simulink model "lab4"  (R2024a)
settings: Solver=VariableStepAuto  StartTime=0.0  StopTime=1  RelTol=1e-3
model workspace (MAT data in the model file):
  ampl = 1
  delta_f = 100
  delta_fc = 4000
  fd = 1024000
undefined symbols (not defined in the file): fdesignblkfcn, gcbh
libraries: dsparch4 x13, commanapbnd3 x13, dspsrcs4 x12, dspfdesign x1
settings Model: Creator=Egor Masterskikh  LastModifiedBy=Egor Masterskikh

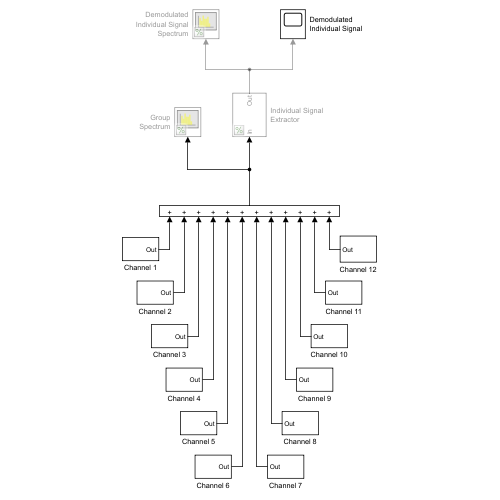
[thumbnail: Simulink's stored preview of the top-level diagram]
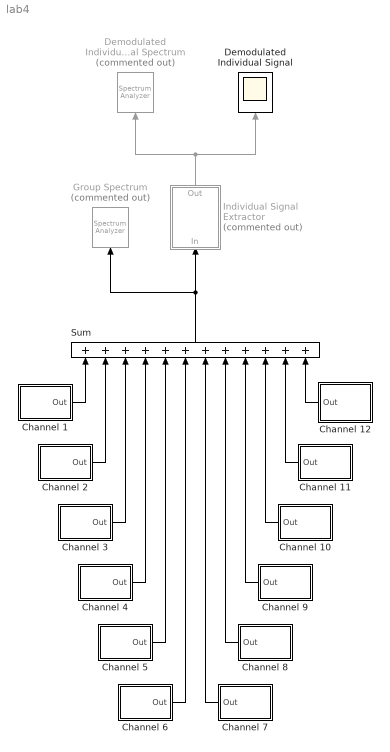
== system lab4 ==
  Channel 1 : Subsystem  mask{f=900, fc=64000}
      mask prompts: f "Frequency (Hz)"; fc "Carrier frequency (Hz)"
  Channel 10 : Subsystem  mask{f=1800, fc=100000}
      mask prompts: f "Frequency (Hz)"; fc "Carrier frequency (Hz)"
  Channel 11 : Subsystem  mask{f=1900, fc=104000}
      mask prompts: f "Frequency (Hz)"; fc "Carrier frequency (Hz)"
  Channel 12 : Subsystem  mask{f=2000, fc=108000}
      mask prompts: f "Frequency (Hz)"; fc "Carrier frequency (Hz)"
  Channel 2 : Subsystem  mask{f=1000, fc=68000}
      mask prompts: f "Frequency (Hz)"; fc "Carrier frequency (Hz)"
  Channel 3 : Subsystem  mask{f=1100, fc=72000}
      mask prompts: f "Frequency (Hz)"; fc "Carrier frequency (Hz)"
  Channel 4 : Subsystem  mask{f=1200, fc=76000}
      mask prompts: f "Frequency (Hz)"; fc "Carrier frequency (Hz)"
  Channel 5 : Subsystem  mask{f=1300, fc=80000}
      mask prompts: f "Frequency (Hz)"; fc "Carrier frequency (Hz)"
  Channel 6 : Subsystem  mask{f=1400, fc=84000}
      mask prompts: f "Frequency (Hz)"; fc "Carrier frequency (Hz)"
  Channel 7 : Subsystem  mask{f=1500, fc=88000}
      mask prompts: f "Frequency (Hz)"; fc "Carrier frequency (Hz)"
  Channel 8 : Subsystem  mask{f=1600, fc=92000}
      mask prompts: f "Frequency (Hz)"; fc "Carrier frequency (Hz)"
  Channel 9 : Subsystem  mask{f=1700, fc=96000}
      mask prompts: f "Frequency (Hz)"; fc "Carrier frequency (Hz)"
  Demodulated Individual Signal : Scope
  Demodulated Individual Signal Spectrum : SpectrumAnalyzer  Commented=on  WindowPosition=[154.000000,73.000000,765.000000,744.000000,]  ScopeFrameLocation=window  SampleRate=44.1e3  PlotAsTwoSidedSpectrum=off  FrequencySpan=Start and stop frequencies  StartFrequency=50  YLimits=[-52.2671399,38.98350768]  SelectedToolstripTab=spectrumAnalyzerToolstrip.estimationTab
  Group Spectrum : SpectrumAnalyzer  Commented=on  WindowPosition=[318.000000,220.000000,765.000000,500.000000,]  ScopeFrameLocation=window  SampleRate=44.1e3  PlotAsTwoSidedSpectrum=off  StartFrequency=20  StopFrequency=20e3  YLimits=[-282.95043207,54.73793571]
  Individual Signal Extractor : Subsystem  Commented=on  mask{ch_num=1, fc=64000, f_cutoff=64100}
      mask prompts: ch_num "Extracted channel number"; fc "Carrier frequency (Hz)"; f_cutoff "Cutoff frequency (Hz)"
  Sum : Sum  Inputs=++++++++++++
  wires:
  Sum/1 -> Group Spectrum/1, Individual Signal Extractor/1(In)
  Channel 1/1(Out) -> Sum/1
  Individual Signal Extractor/1(Out) -> Demodulated Individual Signal/1, Demodulated Individual Signal Spectrum/1
  Channel 12/1(Out) -> Sum/12
  Channel 2/1(Out) -> Sum/2
  Channel 3/1(Out) -> Sum/3
  Channel 4/1(Out) -> Sum/4
  Channel 11/1(Out) -> Sum/11
  Channel 10/1(Out) -> Sum/10
  Channel 9/1(Out) -> Sum/9
  Channel 5/1(Out) -> Sum/5
  Channel 8/1(Out) -> Sum/8
  Channel 6/1(Out) -> Sum/6
  Channel 7/1(Out) -> Sum/7

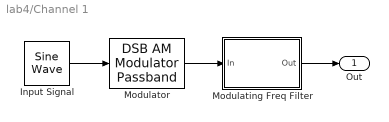
== system lab4/Channel 1 ==
  Input Signal : dspsrcs4/Sine Wave  Amplitude=ampl  Frequency=f  Phase=0  SampleMode=Discrete  OutComplex=Real  CompMethod=Trigonometric fcn  TableSize=Speed  SampleTime=1 / fd  SamplesPerFrame=1  ResetState=Restart at time zero  OutputFrames=off  dataType=double  wordLen=16  udDataType=sfix(16)  fracBitsMode=Best precision  numFracBits=15  OutDataTypeStr=double  LastOutDataTypeStr=double
  Modulating Freq Filter : Subsystem  DialogController=fdesignblkfcn  InitFcn=fdesignblkfcn(gcbh, {'InitFcn'});  mask(Bandpass Filter){}
      mask help: dsp:DSPFilterDesignBlockDialog:BandpassFdesign_MaskDesc
      settings: CopyFcn=fdesignblkfcn(gcbh, {'CopyFcn'});
      mask Help: helpview(mapfilelocation('dsp'), 'dspbandpassfilter');
      mask Display: disp('Bandpass');
  Modulator : commanapbnd3/DSB AM Modulator Passband  Fc=fc  Ph=0  Offset=ampl
  Out : Outport
  wires:
  Modulator/1 -> Modulating Freq Filter/1(In)
  Input Signal/1 -> Modulator/1
  Modulating Freq Filter/1(Out) -> Out/1

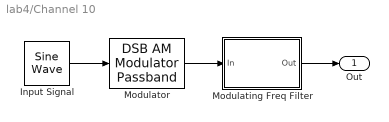
== system lab4/Channel 10 ==
  Input Signal : dspsrcs4/Sine Wave  Amplitude=ampl  Frequency=f  Phase=0  SampleMode=Discrete  OutComplex=Real  CompMethod=Trigonometric fcn  TableSize=Speed  SampleTime=1 / fd  SamplesPerFrame=1  ResetState=Restart at time zero  OutputFrames=off  dataType=double  wordLen=16  udDataType=sfix(16)  fracBitsMode=Best precision  numFracBits=15  OutDataTypeStr=double  LastOutDataTypeStr=double
  Modulating Freq Filter : Subsystem  DialogController=fdesignblkfcn  InitFcn=fdesignblkfcn(gcbh, {'InitFcn'});  mask(Bandpass Filter){}
      mask help: dsp:DSPFilterDesignBlockDialog:BandpassFdesign_MaskDesc
      settings: CopyFcn=fdesignblkfcn(gcbh, {'CopyFcn'});
      mask Help: helpview(mapfilelocation('dsp'), 'dspbandpassfilter');
      mask Display: disp('Bandpass');
  Modulator : commanapbnd3/DSB AM Modulator Passband  Fc=fc  Ph=0  Offset=ampl
  Out : Outport
  wires:
  Modulator/1 -> Modulating Freq Filter/1(In)
  Input Signal/1 -> Modulator/1
  Modulating Freq Filter/1(Out) -> Out/1

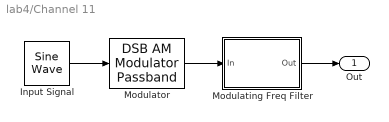
== system lab4/Channel 11 ==
  Input Signal : dspsrcs4/Sine Wave  Amplitude=ampl  Frequency=f  Phase=0  SampleMode=Discrete  OutComplex=Real  CompMethod=Trigonometric fcn  TableSize=Speed  SampleTime=1 / fd  SamplesPerFrame=1  ResetState=Restart at time zero  OutputFrames=off  dataType=double  wordLen=16  udDataType=sfix(16)  fracBitsMode=Best precision  numFracBits=15  OutDataTypeStr=double  LastOutDataTypeStr=double
  Modulating Freq Filter : Subsystem  DialogController=fdesignblkfcn  InitFcn=fdesignblkfcn(gcbh, {'InitFcn'});  mask(Bandpass Filter){}
      mask help: dsp:DSPFilterDesignBlockDialog:BandpassFdesign_MaskDesc
      settings: CopyFcn=fdesignblkfcn(gcbh, {'CopyFcn'});
      mask Help: helpview(mapfilelocation('dsp'), 'dspbandpassfilter');
      mask Display: disp('Bandpass');
  Modulator : commanapbnd3/DSB AM Modulator Passband  Fc=fc  Ph=0  Offset=ampl
  Out : Outport
  wires:
  Modulator/1 -> Modulating Freq Filter/1(In)
  Input Signal/1 -> Modulator/1
  Modulating Freq Filter/1(Out) -> Out/1

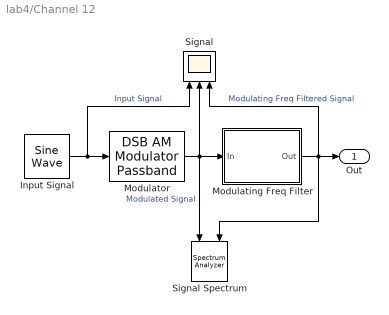
== system lab4/Channel 12 ==
  Input Signal : dspsrcs4/Sine Wave  Amplitude=ampl  Frequency=f  Phase=0  SampleMode=Discrete  OutComplex=Real  CompMethod=Trigonometric fcn  TableSize=Speed  SampleTime=1 / fd  SamplesPerFrame=1  ResetState=Restart at time zero  OutputFrames=off  dataType=double  wordLen=16  udDataType=sfix(16)  fracBitsMode=Best precision  numFracBits=15  OutDataTypeStr=double  LastOutDataTypeStr=double
  Modulating Freq Filter : Subsystem  DialogController=fdesignblkfcn  InitFcn=fdesignblkfcn(gcbh, {'InitFcn'});  mask(Bandpass Filter){}
      mask help: dsp:DSPFilterDesignBlockDialog:BandpassFdesign_MaskDesc
      settings: CopyFcn=fdesignblkfcn(gcbh, {'CopyFcn'});
      mask Help: helpview(mapfilelocation('dsp'), 'dspbandpassfilter');
      mask Display: disp('Bandpass');
  Modulator : commanapbnd3/DSB AM Modulator Passband  Fc=fc  Ph=0  Offset=ampl
  Signal : Scope  NumInputPorts=3
  Signal Spectrum : SpectrumAnalyzer  NumInputPorts=2  WindowPosition=[625.000000,219.000000,459.000000,419.000000,]  Visible=on  ScopeFrameLocation=window  SampleRate=1024000  PlotAsTwoSidedSpectrum=off  FrequencySpan=Start and stop frequencies  StartFrequency=102000  StopFrequency=116000  YLimits=[-95.72814975,34.95307911]  ShowLegend=on  SelectedToolstripTab=spectrumAnalyzerToolstrip.estimationTab
  Out : Outport
  wires:
  Modulator/1 -> Signal Spectrum/1, Signal/2, Modulating Freq Filter/1(In)  "Modulated Signal"
  Input Signal/1 -> Modulator/1, Signal/1  "Input Signal"
  Modulating Freq Filter/1(Out) -> Signal/3, Signal Spectrum/2, Out/1  "Modulating Freq Filtered Signal"

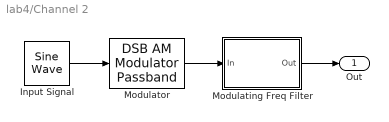
== system lab4/Channel 2 ==
  Input Signal : dspsrcs4/Sine Wave  Amplitude=ampl  Frequency=f  Phase=0  SampleMode=Discrete  OutComplex=Real  CompMethod=Trigonometric fcn  TableSize=Speed  SampleTime=1 / fd  SamplesPerFrame=1  ResetState=Restart at time zero  OutputFrames=off  dataType=double  wordLen=16  udDataType=sfix(16)  fracBitsMode=Best precision  numFracBits=15  OutDataTypeStr=double  LastOutDataTypeStr=double
  Modulating Freq Filter : Subsystem  DialogController=fdesignblkfcn  InitFcn=fdesignblkfcn(gcbh, {'InitFcn'});  mask(Bandpass Filter){}
      mask help: dsp:DSPFilterDesignBlockDialog:BandpassFdesign_MaskDesc
      settings: CopyFcn=fdesignblkfcn(gcbh, {'CopyFcn'});
      mask Help: helpview(mapfilelocation('dsp'), 'dspbandpassfilter');
      mask Display: disp('Bandpass');
  Modulator : commanapbnd3/DSB AM Modulator Passband  Fc=fc  Ph=0  Offset=ampl
  Out : Outport
  wires:
  Modulator/1 -> Modulating Freq Filter/1(In)
  Input Signal/1 -> Modulator/1
  Modulating Freq Filter/1(Out) -> Out/1

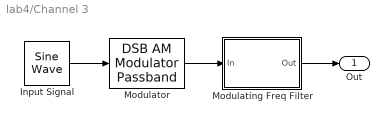
== system lab4/Channel 3 ==
  Input Signal : dspsrcs4/Sine Wave  Amplitude=ampl  Frequency=f  Phase=0  SampleMode=Discrete  OutComplex=Real  CompMethod=Trigonometric fcn  TableSize=Speed  SampleTime=1 / fd  SamplesPerFrame=1  ResetState=Restart at time zero  OutputFrames=off  dataType=double  wordLen=16  udDataType=sfix(16)  fracBitsMode=Best precision  numFracBits=15  OutDataTypeStr=double  LastOutDataTypeStr=double
  Modulating Freq Filter : Subsystem  DialogController=fdesignblkfcn  InitFcn=fdesignblkfcn(gcbh, {'InitFcn'});  mask(Bandpass Filter){}
      mask help: dsp:DSPFilterDesignBlockDialog:BandpassFdesign_MaskDesc
      settings: CopyFcn=fdesignblkfcn(gcbh, {'CopyFcn'});
      mask Help: helpview(mapfilelocation('dsp'), 'dspbandpassfilter');
      mask Display: disp('Bandpass');
  Modulator : commanapbnd3/DSB AM Modulator Passband  Fc=fc  Ph=0  Offset=ampl
  Out : Outport
  wires:
  Modulator/1 -> Modulating Freq Filter/1(In)
  Input Signal/1 -> Modulator/1
  Modulating Freq Filter/1(Out) -> Out/1

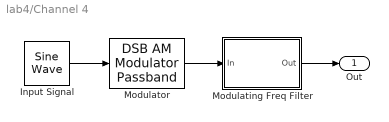
== system lab4/Channel 4 ==
  Input Signal : dspsrcs4/Sine Wave  Amplitude=ampl  Frequency=f  Phase=0  SampleMode=Discrete  OutComplex=Real  CompMethod=Trigonometric fcn  TableSize=Speed  SampleTime=1 / fd  SamplesPerFrame=1  ResetState=Restart at time zero  OutputFrames=off  dataType=double  wordLen=16  udDataType=sfix(16)  fracBitsMode=Best precision  numFracBits=15  OutDataTypeStr=double  LastOutDataTypeStr=double
  Modulating Freq Filter : Subsystem  DialogController=fdesignblkfcn  InitFcn=fdesignblkfcn(gcbh, {'InitFcn'});  mask(Bandpass Filter){}
      mask help: dsp:DSPFilterDesignBlockDialog:BandpassFdesign_MaskDesc
      settings: CopyFcn=fdesignblkfcn(gcbh, {'CopyFcn'});
      mask Help: helpview(mapfilelocation('dsp'), 'dspbandpassfilter');
      mask Display: disp('Bandpass');
  Modulator : commanapbnd3/DSB AM Modulator Passband  Fc=fc  Ph=0  Offset=ampl
  Out : Outport
  wires:
  Modulator/1 -> Modulating Freq Filter/1(In)
  Input Signal/1 -> Modulator/1
  Modulating Freq Filter/1(Out) -> Out/1

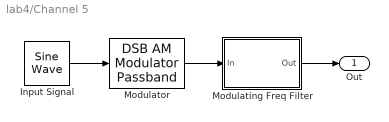
== system lab4/Channel 5 ==
  Input Signal : dspsrcs4/Sine Wave  Amplitude=ampl  Frequency=f  Phase=0  SampleMode=Discrete  OutComplex=Real  CompMethod=Trigonometric fcn  TableSize=Speed  SampleTime=1 / fd  SamplesPerFrame=1  ResetState=Restart at time zero  OutputFrames=off  dataType=double  wordLen=16  udDataType=sfix(16)  fracBitsMode=Best precision  numFracBits=15  OutDataTypeStr=double  LastOutDataTypeStr=double
  Modulating Freq Filter : Subsystem  DialogController=fdesignblkfcn  InitFcn=fdesignblkfcn(gcbh, {'InitFcn'});  mask(Bandpass Filter){}
      mask help: dsp:DSPFilterDesignBlockDialog:BandpassFdesign_MaskDesc
      settings: CopyFcn=fdesignblkfcn(gcbh, {'CopyFcn'});
      mask Help: helpview(mapfilelocation('dsp'), 'dspbandpassfilter');
      mask Display: disp('Bandpass');
  Modulator : commanapbnd3/DSB AM Modulator Passband  Fc=fc  Ph=0  Offset=ampl
  Out : Outport
  wires:
  Modulator/1 -> Modulating Freq Filter/1(In)
  Input Signal/1 -> Modulator/1
  Modulating Freq Filter/1(Out) -> Out/1

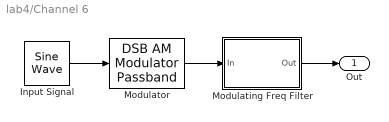
== system lab4/Channel 6 ==
  Input Signal : dspsrcs4/Sine Wave  Amplitude=ampl  Frequency=f  Phase=0  SampleMode=Discrete  OutComplex=Real  CompMethod=Trigonometric fcn  TableSize=Speed  SampleTime=1 / fd  SamplesPerFrame=1  ResetState=Restart at time zero  OutputFrames=off  dataType=double  wordLen=16  udDataType=sfix(16)  fracBitsMode=Best precision  numFracBits=15  OutDataTypeStr=double  LastOutDataTypeStr=double
  Modulating Freq Filter : Subsystem  DialogController=fdesignblkfcn  InitFcn=fdesignblkfcn(gcbh, {'InitFcn'});  mask(Bandpass Filter){}
      mask help: dsp:DSPFilterDesignBlockDialog:BandpassFdesign_MaskDesc
      settings: CopyFcn=fdesignblkfcn(gcbh, {'CopyFcn'});
      mask Help: helpview(mapfilelocation('dsp'), 'dspbandpassfilter');
      mask Display: disp('Bandpass');
  Modulator : commanapbnd3/DSB AM Modulator Passband  Fc=fc  Ph=0  Offset=ampl
  Out : Outport
  wires:
  Modulator/1 -> Modulating Freq Filter/1(In)
  Input Signal/1 -> Modulator/1
  Modulating Freq Filter/1(Out) -> Out/1

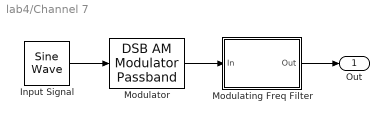
== system lab4/Channel 7 ==
  Input Signal : dspsrcs4/Sine Wave  Amplitude=ampl  Frequency=f  Phase=0  SampleMode=Discrete  OutComplex=Real  CompMethod=Trigonometric fcn  TableSize=Speed  SampleTime=1 / fd  SamplesPerFrame=1  ResetState=Restart at time zero  OutputFrames=off  dataType=double  wordLen=16  udDataType=sfix(16)  fracBitsMode=Best precision  numFracBits=15  OutDataTypeStr=double  LastOutDataTypeStr=double
  Modulating Freq Filter : Subsystem  DialogController=fdesignblkfcn  InitFcn=fdesignblkfcn(gcbh, {'InitFcn'});  mask(Bandpass Filter){}
      mask help: dsp:DSPFilterDesignBlockDialog:BandpassFdesign_MaskDesc
      settings: CopyFcn=fdesignblkfcn(gcbh, {'CopyFcn'});
      mask Help: helpview(mapfilelocation('dsp'), 'dspbandpassfilter');
      mask Display: disp('Bandpass');
  Modulator : commanapbnd3/DSB AM Modulator Passband  Fc=fc  Ph=0  Offset=ampl
  Out : Outport
  wires:
  Modulator/1 -> Modulating Freq Filter/1(In)
  Input Signal/1 -> Modulator/1
  Modulating Freq Filter/1(Out) -> Out/1

== system lab4/Channel 8 ==
  Input Signal : dspsrcs4/Sine Wave  Amplitude=ampl  Frequency=f  Phase=0  SampleMode=Discrete  OutComplex=Real  CompMethod=Trigonometric fcn  TableSize=Speed  SampleTime=1 / fd  SamplesPerFrame=1  ResetState=Restart at time zero  OutputFrames=off  dataType=double  wordLen=16  udDataType=sfix(16)  fracBitsMode=Best precision  numFracBits=15  OutDataTypeStr=double  LastOutDataTypeStr=double
  Modulating Freq Filter : Subsystem  DialogController=fdesignblkfcn  InitFcn=fdesignblkfcn(gcbh, {'InitFcn'});  mask(Bandpass Filter){}
      mask help: dsp:DSPFilterDesignBlockDialog:BandpassFdesign_MaskDesc
      settings: CopyFcn=fdesignblkfcn(gcbh, {'CopyFcn'});
      mask Help: helpview(mapfilelocation('dsp'), 'dspbandpassfilter');
      mask Display: disp('Bandpass');
  Modulator : commanapbnd3/DSB AM Modulator Passband  Fc=fc  Ph=0  Offset=ampl
  Out : Outport
  wires:
  Modulator/1 -> Modulating Freq Filter/1(In)
  Input Signal/1 -> Modulator/1
  Modulating Freq Filter/1(Out) -> Out/1

== system lab4/Channel 9 ==
  Input Signal : dspsrcs4/Sine Wave  Amplitude=ampl  Frequency=f  Phase=0  SampleMode=Discrete  OutComplex=Real  CompMethod=Trigonometric fcn  TableSize=Speed  SampleTime=1 / fd  SamplesPerFrame=1  ResetState=Restart at time zero  OutputFrames=off  dataType=double  wordLen=16  udDataType=sfix(16)  fracBitsMode=Best precision  numFracBits=15  OutDataTypeStr=double  LastOutDataTypeStr=double
  Modulating Freq Filter : Subsystem  DialogController=fdesignblkfcn  InitFcn=fdesignblkfcn(gcbh, {'InitFcn'});  mask(Bandpass Filter){}
      mask help: dsp:DSPFilterDesignBlockDialog:BandpassFdesign_MaskDesc
      settings: CopyFcn=fdesignblkfcn(gcbh, {'CopyFcn'});
      mask Help: helpview(mapfilelocation('dsp'), 'dspbandpassfilter');
      mask Display: disp('Bandpass');
  Modulator : commanapbnd3/DSB AM Modulator Passband  Fc=fc  Ph=0  Offset=ampl
  Out : Outport
  wires:
  Modulator/1 -> Modulating Freq Filter/1(In)
  Input Signal/1 -> Modulator/1
  Modulating Freq Filter/1(Out) -> Out/1

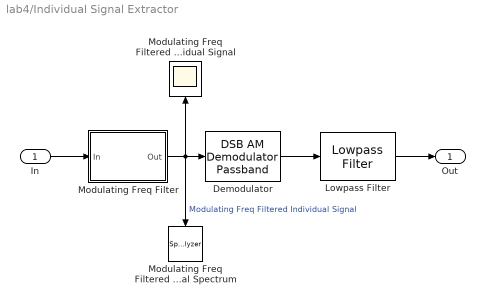
== system lab4/Individual Signal Extractor ==
  In : Inport
  Demodulator : commanapbnd3/DSB AM Demodulator Passband  Fc=fc  Ph=0  method=Butterworth  n=2  cf=f_cutoff  Rp=0.1  Rs=50  Offset=ampl
  Lowpass Filter : dspfdesign/Lowpass Filter  FilterType=IIR  DesignForMinimumOrder=on  FilterOrder=50  PassbandFrequency=fc - delta_fc  StopbandFrequency=fc  PassbandRipple=0.1  StopbandAttenuation=80  SampleRateMode=Specify on dialog  SampleRate=fd  SimulateUsing=Interpreted execution  roundingMode=Floor  coeffsDataTypeStr=fixdt(1,16)
  Modulating Freq Filter : Subsystem  DialogController=fdesignblkfcn  InitFcn=fdesignblkfcn(gcbh, {'InitFcn'});  mask(Bandpass Filter){}
      mask help: dsp:DSPFilterDesignBlockDialog:BandpassFdesign_MaskDesc
      settings: CopyFcn=fdesignblkfcn(gcbh, {'CopyFcn'});
      mask Help: helpview(mapfilelocation('dsp'), 'dspbandpassfilter');
      mask Display: disp('Bandpass');
  Modulating Freq Filtered Individual Signal : Scope
  Modulating Freq Filtered Individual Signal Spectrum : SpectrumAnalyzer  WindowPosition=[105.000000,360.000000,765.000000,500.000000,]  ScopeFrameLocation=window  SampleRate=44.1e3  PlotAsTwoSidedSpectrum=off  FrequencyScale=Log  StartFrequency=20  StopFrequency=20e3  YLimits=[-284.08053671,64.89783602]  SelectedToolstripTab=spectrumAnalyzerToolstrip.spectrumTab
  Out : Outport
  wires:
  Modulating Freq Filter/1(Out) -> Modulating Freq Filtered Individual Signal/1, Modulating Freq Filtered Individual Signal Spectrum/1, Demodulator/1  "Modulating Freq Filtered Individual Signal"
  In/1 -> Modulating Freq Filter/1(In)
  Demodulator/1 -> Lowpass Filter/1
  Lowpass Filter/1 -> Out/1

== system lab4/Channel 1/Modulating Freq Filter ==
  In : Inport
  Generated Filter Block : dsparch4/Biquad Filter  Tag=BlockMethodSubSystem  FilterSource=Dialog parameters  CoeffSource=Specify via dialog  FilterObject=BQF  IIRFiltStruct=Direct form II  BiQuadCoeffs=[0.000447834192739895044 0 -0.000447834192739895044 1 -1.84342145835843008 0.999668405594225651;0.000352702272994555224 0 -0.000352702272994555224 1 -1.84297530266396015 0.99966795227800076;0.000393389037410715866 0 -0.000393389037410715866 1 -1.84295972447575496 0.999351069372707124;0.000271522397118558259 0 -0.000271522397118558259 1 -1.84285253444748021 0.99935085656781808;0.000439928533426870458 0 -0.000439928533426870458 1 -1.8431609620298508 0.999463406116796627;0.000179968694146031232 0 -0.000179968694146031232 1 -1.8428580048816825 0.999462908410175377;0.000433029410195073577 0 -0.000433029410195073577 1 -1.84369625970029016 0.999930675836544713;0.000269558668079343837 0 -0.000269558668079343837 1 -1.8431842180074598 0.999930566975026469;0.000434295423850435938 0 -0.000434295423850435938 1 -1.84328645928743917 0.999556221907486164;0.000385090966757165032 0 -0.000385090966757165032 1 -1.84290350897479316 0.999555701394280849;0.000303547956367676715 0 -0.000303547956367676715 1 -1.8428927773742525 0.999336467904331727;0.000418382354530299778 0 -0.000418382354530299778 1 -1.84305044171901544 0.999394010334468064;0.000191838924433208831 0 -0.000191838924433208831 1 -1.8428407671553253 0.999393621449692682;0.00048034125864483652 0 -0.00048034125864483652 1 -1.84356007278210687 0.999795064162199099;1.28986266810011485 0 -1.28986266810011485 1 -1.84307025531527069 0.999794756459478462]  ScaleValues=[0.00016526438313770015;1;1;1;1;1;1;1;1;1;1;1;1;1;1;1]  IC=0  ICnum=0  ICden=0  a0Flag=Warning  optimizeScaleValues=off  ScaleValueMode=Specify via input port (g)  roundingMode=Floor  overflowMode=off  scaleValueFracLength=14  denProdOutputFracLength=30  denAccumFracLength=30  secondMemoryFracLength=15
  Out : Outport  VectorParamsAs1DForOutWhenUnconnected=off
  wires:
  In/1 -> Generated Filter Block/1
  Generated Filter Block/1 -> Out/1

== system lab4/Channel 10/Modulating Freq Filter ==
  In : Inport
  Generated Filter Block : dsparch4/Biquad Filter  Tag=BlockMethodSubSystem  FilterSource=Dialog parameters  CoeffSource=Specify via dialog  FilterObject=BQF  IIRFiltStruct=Direct form II  BiQuadCoeffs=[0.000617160997669246214 0 -0.000617160997669246214 1 -1.62241794392615835 0.999668235825714513;0.000370688453778296825 0 -0.000370688453778296825 1 -1.621745367817095 0.999667971176494863;0.000324715649364414668 0 -0.000324715649364414668 1 -1.62190515232035515 0.999350877580746921;0.000381943679476062314 0 -0.000381943679476062314 1 -1.62174365944132948 0.99935075330712575;0.000293479154670948602 0 -0.000293479154670948602 1 -1.62214364749491913 0.999463180522007555;0.000102390689493418523 0 -0.000102390689493418523 1 -1.62168711613890837 0.99946288994218524;0.000638143829259384663 0 -0.000638143829259384663 1 -1.62268068636250073 0.999930637405414213;0.000229978456795020767 0 -0.000229978456795020767 1 -1.62190841043584166 0.999930573857458205;0.00059646218730135018 0 -0.00059646218730135018 1 -1.62227922962667037 0.999556012651295678;0.000435265460218773681 0 -0.000435265460218773681 1 -1.6217020556082069 0.999555708769626738;0.000361638672273185806 0 -0.000361638672273185806 1 -1.62181265288937149 0.99933631708436399;0.000315644330992207345 0 -0.000315644330992207345 1 -1.62201711391125469 0.999393791619882288;0.000174690159282568197 0 -0.000174690159282568197 1 -1.62170119246115485 0.999393564586653849;0.00060369892230943635 0 -0.00060369892230943635 1 -1.62255373803222858 0.999794953506548456;0.854898081973351931 0 -0.854898081973351931 1 -1.6218151679562347 0.999794773860514407]  ScaleValues=[0.000195243173911168887;1;1;1;1;1;1;1;1;1;1;1;1;1;1;1]  IC=0  ICnum=0  ICden=0  a0Flag=Warning  optimizeScaleValues=off  ScaleValueMode=Specify via input port (g)  roundingMode=Floor  overflowMode=off  scaleValueFracLength=14  denProdOutputFracLength=30  denAccumFracLength=30  secondMemoryFracLength=15
  Out : Outport  VectorParamsAs1DForOutWhenUnconnected=off
  wires:
  In/1 -> Generated Filter Block/1
  Generated Filter Block/1 -> Out/1

== system lab4/Channel 11/Modulating Freq Filter ==
  In : Inport
  Generated Filter Block : dsparch4/Biquad Filter  Tag=BlockMethodSubSystem  FilterSource=Dialog parameters  CoeffSource=Specify via dialog  FilterObject=BQF  IIRFiltStruct=Direct form II  BiQuadCoeffs=[0.000447628501381116086 0 -0.000447628501381116086 1 -1.59250017362264762 0.99966822362923069;0.000352954626275813106 0 -0.000352954626275813106 1 -1.59180435375816853 0.99966797253053219;0.00039345614439857576 0 -0.00039345614439857576 1 -1.59198329056691823 0.999350863781894083;0.000271644733088461222 0 -0.000271644733088461222 1 -1.59181622174333626 0.999350745901675053;0.000439944764822964727 0 -0.000439944764822964727 1 -1.59222520465960216 0.999463164309352559;0.000180075495854922958 0 -0.000180075495854922958 1 -1.59175290520271417 0.999462888614995992;0.00043288613625754621 0 -0.00043288613625754621 1 -1.59276072419261983 0.999930634647579142;0.000269755438726646424 0 -0.000269755438726646424 1 -1.59196173881381497 0.999930574348017798;0.000434143116867879856 0 -0.000434143116867879856 1 -1.59236148543245948 0.999555997613725822;0.000385313111562148275 0 -0.000385313111562148275 1 -1.59176437113480529 0.999555709298804662;0.000303665389116391452 0 -0.000303665389116391452 1 -1.59188821983248996 0.999336306245515615;0.000418424444953989863 0 -0.000418424444953989863 1 -1.59209727832879144 0.999393775914295901;0.000191949844049738104 0 -0.000191949844049738104 1 -1.59177044744471052 0.999393560487543686;0.000480297562160769296 0 -0.000480297562160769296 1 -1.59263521764399663 0.99979494555622539;0.826582306747762674 0 -0.826582306747762674 1 -1.59187111381208402 0.999794775108989731]  ScaleValues=[0.000258032713105099112;1;1;1;1;1;1;1;1;1;1;1;1;1;1;1]  IC=0  ICnum=0  ICden=0  a0Flag=Warning  optimizeScaleValues=off  ScaleValueMode=Specify via input port (g)  roundingMode=Floor  overflowMode=off  scaleValueFracLength=14  denProdOutputFracLength=30  denAccumFracLength=30  secondMemoryFracLength=15
  Out : Outport  VectorParamsAs1DForOutWhenUnconnected=off
  wires:
  In/1 -> Generated Filter Block/1
  Generated Filter Block/1 -> Out/1

== system lab4/Channel 12/Modulating Freq Filter ==
  In : Inport
  Generated Filter Block : dsparch4/Biquad Filter  Tag=BlockMethodSubSystem  FilterSource=Dialog parameters  CoeffSource=Specify via dialog  FilterObject=BQF  IIRFiltStruct=Direct form II  BiQuadCoeffs=[0.000575044595653252341 0 -0.000575044595653252341 1 -1.56157458163508611 0.999668212209986029;0.000331837978043018076 0 -0.000331837978043018076 1 -1.5608559572839158 0.999667973801524279;0.000331870744427895472 0 -0.000331870744427895472 1 -1.56105393440636386 0.999350850877665398;0.000331826647990149566 0 -0.000331826647990149566 1 -1.56088139478725729 0.999350738959238427;0.000331919314966763464 0 -0.000331919314966763464 1 -1.56129911447708203 0.999463149131103346;0.000331872132384747841 0 -0.000331872132384747841 1 -1.56081134462767901 0.999462887376403875;0.000332029027386733088 0 -0.000332029027386733088 1 -1.5618327746913887 0.999930632063309566;0.000331829796170876471 0 -0.000331829796170876471 1 -1.56100758524146821 0.999930574810165895;0.000331946973926153927 0 -0.000331946973926153927 1 -1.56143600756156697 0.999555983540826753;0.000331851954888435499 0 -0.000331851954888435499 1 -1.56081932960614567 0.999555709792220193;0.000331829414474926288 0 -0.000331829414474926288 1 -1.56095635226284224 0.999336296100635679;0.000331893530768644573 0 -0.000331893530768644573 1 -1.56116987630114168 0.999393761190399799;0.000331853043227300058 0 -0.000331853043227300058 1 -1.56083234192654929 0.999393556674763817;0.000332003053029892746 0 -0.000332003053029892746 1 -1.56170878976648364 0.999794938111094544;0.800179900857727611 0 -0.800179900857727611 1 -1.5609196350121648 0.999794776281361042]  ScaleValues=[0.000239410766507700559;1;1;1;1;1;1;1;1;1;1;1;1;1;1;1]  IC=0  ICnum=0  ICden=0  a0Flag=Warning  optimizeScaleValues=off  ScaleValueMode=Specify via input port (g)  InputProcessing=Columns as channels (frame based)  roundingMode=Floor  overflowMode=off  scaleValueFracLength=14  denProdOutputFracLength=30  denAccumFracLength=30  secondMemoryFracLength=15
  Out : Outport  VectorParamsAs1DForOutWhenUnconnected=off
  wires:
  In/1 -> Generated Filter Block/1
  Generated Filter Block/1 -> Out/1

== system lab4/Channel 2/Modulating Freq Filter ==
  In : Inport
  Generated Filter Block : dsparch4/Biquad Filter  Tag=BlockMethodSubSystem  FilterSource=Dialog parameters  CoeffSource=Specify via dialog  FilterObject=BQF  IIRFiltStruct=Direct form II  BiQuadCoeffs=[0.000575123834762801284 0 -0.000575123834762801284 1 -1.82334579078760206 0.999668378524630641;0.000331751411565755247 0 -0.000331751411565755247 1 -1.822873139200621 0.999667955296015376;0.00033180956165842682 0 -0.00033180956165842682 1 -1.82287716004175349 0.999351038794542013;0.00033171686748468209 0 -0.00033171686748468209 1 -1.82276361736392323 0.999350840108934046;0.000331881326789953133 0 -0.000331881326789953133 1 -1.82308308248949658 0.99946337015809561;0.000331737447761673359 0 -0.000331737447761673359 1 -1.82276215740922654 0.999462905460592799;0.000332015884975879591 0 -0.000332015884975879591 1 -1.82361994698937968 0.999930669708638642;0.000331710522637327656 0 -0.000331710522637327656 1 -1.82307744502172975 0.999930568073465809;0.000331918475081411225 0 -0.000331918475081411225 1 -1.82321002989389092 0.999556188547201629;0.000331778086058353281 0 -0.000331778086058353281 1 -1.82280435374728755 0.99955570257088755;0.000331730704711393376 0 -0.000331730704711393376 1 -1.82280718166096101 0.999336443860735169;0.000331844492539018336 0 -0.000331844492539018336 1 -1.82297048708287468 0.999393975463013118;0.000331721035237542801 0 -0.000331721035237542801 1 -1.82274838263030392 0.99939361238877833;0.000331987253053051012 0 -0.000331987253053051012 1 -1.82348444496896045 0.999795046520630004;1.21700946042950342 0 -1.21700946042950342 1 -1.82296551483073754 0.999794759234470698]  ScaleValues=[0.000157320058972569901;1;1;1;1;1;1;1;1;1;1;1;1;1;1;1]  IC=0  ICnum=0  ICden=0  a0Flag=Warning  optimizeScaleValues=off  ScaleValueMode=Specify via input port (g)  roundingMode=Floor  overflowMode=off  scaleValueFracLength=14  denProdOutputFracLength=30  denAccumFracLength=30  secondMemoryFracLength=15
  Out : Outport  VectorParamsAs1DForOutWhenUnconnected=off
  wires:
  In/1 -> Generated Filter Block/1
  Generated Filter Block/1 -> Out/1

== system lab4/Channel 3/Modulating Freq Filter ==
  In : Inport
  Generated Filter Block : dsparch4/Biquad Filter  Tag=BlockMethodSubSystem  FilterSource=Dialog parameters  CoeffSource=Specify via dialog  FilterObject=BQF  IIRFiltStruct=Direct form II  BiQuadCoeffs=[0.000543679286184926705 0 -0.000543679286184926705 1 -1.80211621175615688 0.999668354319149688;0.000362227721623832155 0 -0.000362227721623832155 1 -1.80161735989500915 0.999667957989932243;0.000383816471205811606 0 -0.000383816471205811606 1 -1.80164098117838867 0.999351011473250672;0.000311136349129568785 0 -0.000311136349129568785 1 -1.80152115595372497 0.999350825360612705;0.000384039083856398795 0 -0.000384039083856398795 1 -1.80185145878272457 0.999463337983039435;0.000138540613445897254 0 -0.000138540613445897254 1 -1.80151276501151081 0.999462902836348532;0.000561574074871164187 0 -0.000561574074871164187 1 -1.80238954688484965 0.999930664233239064;0.000222539328182694241 0 -0.000222539328182694241 1 -1.80181692712690911 0.999930569050549889;0.000526049364986063621 0 -0.000526049364986063621 1 -1.80197977567703926 0.999556158708325038;0.000385766222977939775 0 -0.000385766222977939775 1 -1.80155162642969535 0.999555703624899539;0.000332334777153678155 0 -0.000332334777153678155 1 -1.80156801498856156 0.999336422356312148;0.000382298111173136606 0 -0.000382298111173136606 1 -1.80173685940791484 0.999393944278271107;0.000165696569004271848 0 -0.000165696569004271848 1 -1.80150246260779134 0.999393604280728542;0.000555570682031914041 0 -0.000555570682031914041 1 -1.8022548168582273 0.999795030745955104;1.15355396819730882 0 -1.15355396819730882 1 -1.80170710006907386 0.999794761712590185]  ScaleValues=[0.000152098338985973494;1;1;1;1;1;1;1;1;1;1;1;1;1;1;1]  IC=0  ICnum=0  ICden=0  a0Flag=Warning  optimizeScaleValues=off  ScaleValueMode=Specify via input port (g)  roundingMode=Floor  overflowMode=off  scaleValueFracLength=14  denProdOutputFracLength=30  denAccumFracLength=30  secondMemoryFracLength=15
  Out : Outport  VectorParamsAs1DForOutWhenUnconnected=off
  wires:
  In/1 -> Generated Filter Block/1
  Generated Filter Block/1 -> Out/1

== system lab4/Channel 4/Modulating Freq Filter ==
  In : Inport
  Generated Filter Block : dsparch4/Biquad Filter  Tag=BlockMethodSubSystem  FilterSource=Dialog parameters  CoeffSource=Specify via dialog  FilterObject=BQF  IIRFiltStruct=Direct form II  BiQuadCoeffs=[0.000430987441720486657 0 -0.000430987441720486657 1 -1.77974615603631214 0.999668332511227109;0.000337773398596887464 0 -0.000337773398596887464 1 -1.77922141665462208 0.999667960420842605;0.000355750681035559707 0 -0.000355750681035559707 1 -1.77926462667238594 0.999350986819394382;0.000293305561417332001 0 -0.000293305561417332001 1 -1.7791385934601216 0.999350812119327525;0.00038204525803523854 0 -0.00038204525803523854 1 -1.77947952680747812 0.999463309008189138;0.000255667150765867405 0 -0.000255667150765867405 1 -1.77912327546489291 0.999462900464947235;0.000255827519060255744 0 -0.000255827519060255744 1 -1.78001849505125076 0.999930659291301871;0.000446246822731089876 0 -0.000446246822731089876 1 -1.77941611918634224 0.999930569940515435;0.000307346966844950463 0 -0.000307346966844950463 1 -1.77960913175004332 0.999556131832025185;0.000434656597585560958 0 -0.000434656597585560958 1 -1.7791587769435 0.999555704572601789;0.000308609002114123654 0 -0.000308609002114123654 1 -1.77918871826581171 0.99933640298572235;0.000369739619803979196 0 -0.000369739619803979196 1 -1.77936299589204183 0.999393916188880072;0.000259938165928068137 0 -0.000259938165928068137 1 -1.77911645254787376 0.999393596976260734;0.000405671772379941553 0 -0.000405671772379941553 1 -1.77988462340411369 0.999795016528218339;1.0962322580265631 0 -1.0962322580265631 1 -1.77930846461387926 0.999794763953149701]  ScaleValues=[0.000218274896374907315;1;1;1;1;1;1;1;1;1;1;1;1;1;1;1]  IC=0  ICnum=0  ICden=0  a0Flag=Warning  optimizeScaleValues=off  ScaleValueMode=Specify via input port (g)  roundingMode=Floor  overflowMode=off  scaleValueFracLength=14  denProdOutputFracLength=30  denAccumFracLength=30  secondMemoryFracLength=15
  Out : Outport  VectorParamsAs1DForOutWhenUnconnected=off
  wires:
  In/1 -> Generated Filter Block/1
  Generated Filter Block/1 -> Out/1

== system lab4/Channel 5/Modulating Freq Filter ==
  In : Inport
  Generated Filter Block : dsparch4/Biquad Filter  Tag=BlockMethodSubSystem  FilterSource=Dialog parameters  CoeffSource=Specify via dialog  FilterObject=BQF  IIRFiltStruct=Direct form II  BiQuadCoeffs=[0.000617207435201474835 0 -0.000617207435201474835 1 -1.75624978029114898 0.999668312747239995;0.000370681281013267273 0 -0.000370681281013267273 1 -1.75569948289534494 0.999667962618484451;0.000324692912263799889 0 -0.000324692912263799889 1 -1.75576225718202661 0.99935096449479599;0.000381890650090222937 0 -0.000381890650090222937 1 -1.75563009450296059 0.999350800089863656;0.000293463421742333756 0 -0.000293463421742333756 1 -1.75598144428310654 0.999463282743303649;0.000102327475116689655 0 -0.000102327475116689655 1 -1.75560785802595865 0.999462898312713288;0.000638204141767928848 0 -0.000638204141767928848 1 -1.75652094906380718 0.999930654817252629;0.00022993759343581201 0 -0.00022993759343581201 1 -1.75588919767698504 0.999930570741241698;0.000596496062657758393 0 -0.000596496062657758393 1 -1.75611225502637591 0.9995561074651369;0.000435311437114305167 0 -0.000435311437114305167 1 -1.75563997675568073 0.999555705433771702;0.000361537444693739831 0 -0.000361537444693739831 1 -1.75568345402211645 0.999336385425202978;0.000315675877805895642 0 -0.000315675877805895642 1 -1.75586305548204891 0.999393890720734368;0.000174626438472109659 0 -0.000174626438472109659 1 -1.75560451943031737 0.999393590357900208;0.000603775614659415676 0 -0.000603775614659415676 1 -1.75638802150038553 0.999795003645970959;1.04496733799199948 0 -1.04496733799199948 1 -1.75578378356884346 0.999794765977430333]  ScaleValues=[0.000159669346113225461;1;1;1;1;1;1;1;1;1;1;1;1;1;1;1]  IC=0  ICnum=0  ICden=0  a0Flag=Warning  optimizeScaleValues=off  ScaleValueMode=Specify via input port (g)  roundingMode=Floor  overflowMode=off  scaleValueFracLength=14  denProdOutputFracLength=30  denAccumFracLength=30  secondMemoryFracLength=15
  Out : Outport  VectorParamsAs1DForOutWhenUnconnected=off
  wires:
  In/1 -> Generated Filter Block/1
  Generated Filter Block/1 -> Out/1

== system lab4/Channel 6/Modulating Freq Filter ==
  In : Inport
  Generated Filter Block : dsparch4/Biquad Filter  Tag=BlockMethodSubSystem  FilterSource=Dialog parameters  CoeffSource=Specify via dialog  FilterObject=BQF  IIRFiltStruct=Direct form II  BiQuadCoeffs=[0.000447708823283435189 0 -0.000447708823283435189 1 -1.73164195400504006 0.999668294725545525;0.000352856030694655176 0 -0.000352856030694655176 1 -1.73106644466240689 0.999667964622671157;0.000393429928474345358 0 -0.000393429928474345358 1 -1.73114874592209689 0.999350944115155126;0.00027159693164132922 0 -0.00027159693164132922 1 -1.73101053642931624 0.999350789144468066;0.000439938422088532869 0 -0.000439938422088532869 1 -1.73137208170018075 0.999463258790692421;0.00018003375860722439 0 -0.00018003375860722439 1 -1.73098139452280875 0.999462896353765728;0.000432942098717320684 0 -0.000432942098717320684 1 -1.7319117793959462 0.999930650740405436;0.000269678544631130372 0 -0.000269678544631130372 1 -1.7312510517662818 0.999930571468639617;0.000434202606125313312 0 -0.000434202606125313312 1 -1.73150401526998676 0.999556085254387217;0.000385226312499214075 0 -0.000385226312499214075 1 -1.73101010987430959 0.999555706211314621;0.000303619505270350497 0 -0.000303619505270350497 1 -1.73106709742492559 0.999336369413008185;0.000418407996665496858 0 -0.000418407996665496858 1 -1.73125190986496058 0.999393867509420941;0.000191906497272098026 0 -0.000191906497272098026 1 -1.73098154280097694 0.999393584311795258;0.000480314628465448813 0 -0.000480314628465448813 1 -1.73177988088135626 0.99979499190149157;0.999557396456778657 0 -0.999557396456778657 1 -1.73114794471441291 0.999794767821285402]  ScaleValues=[0.000213334008769975144;1;1;1;1;1;1;1;1;1;1;1;1;1;1;1]  IC=0  ICnum=0  ICden=0  a0Flag=Warning  optimizeScaleValues=off  ScaleValueMode=Specify via input port (g)  roundingMode=Floor  overflowMode=off  scaleValueFracLength=14  denProdOutputFracLength=30  denAccumFracLength=30  secondMemoryFracLength=15
  Out : Outport  VectorParamsAs1DForOutWhenUnconnected=off
  wires:
  In/1 -> Generated Filter Block/1
  Generated Filter Block/1 -> Out/1

== system lab4/Channel 7/Modulating Freq Filter ==
  In : Inport
  Generated Filter Block : dsparch4/Biquad Filter  Tag=BlockMethodSubSystem  FilterSource=Dialog parameters  CoeffSource=Specify via dialog  FilterObject=BQF  IIRFiltStruct=Direct form II  BiQuadCoeffs=[0.000575076018320558715 0 -0.000575076018320558715 1 -1.70593825013830491 0.999668278204689509;0.000331803626902497559 0 -0.000331803626902497559 1 -1.70533789113040424 0.999667966460861424;0.000331846470685980325 0 -0.000331846470685980325 1 -1.70543966946330938 0.999350925449355554;0.000331783088542788652 0 -0.000331783088542788652 1 -1.70529549965815796 0.999350779095760977;0.000331904247195227774 0 -0.000331904247195227774 1 -1.70566701289745337 0.999463236835662849;0.000331818683675431264 0 -0.000331818683675431264 1 -1.70525946992595157 0.99946289455662507;0.000332023814705221176 0 -0.000332023814705221176 1 -1.70620656004299009 0.99993064700065748;0.000331782467187776613 0 -0.000331782467187776613 1 -1.70551727385194285 0.999930572138074236;0.000331935669805874338 0 -0.000331935669805874338 1 -1.70579998563100066 0.999556064887378026;0.000331822641296352836 0 -0.000331822641296352836 1 -1.70528476346381952 0.999555706931297472;0.000331790243239466268 0 -0.000331790243239466268 1 -1.70535522685154683 0.999336354735218757;0.000331874074099156242 0 -0.000331874074099156242 1 -1.7055451339901504 0.999393846217573989;0.000331800658232085416 0 -0.000331800658232085416 1 -1.70526310539511416 0.999393578784450232;0.00033199678706248353 0 -0.00033199678706248353 1 -1.70607577478352179 0.999794981128026783;0.957899660493841343 0 -0.957899660493841343 1 -1.70541653900506196 0.999794769519218418]  ScaleValues=[0.000199945103069872852;1;1;1;1;1;1;1;1;1;1;1;1;1;1;1]  IC=0  ICnum=0  ICden=0  a0Flag=Warning  optimizeScaleValues=off  ScaleValueMode=Specify via input port (g)  roundingMode=Floor  overflowMode=off  scaleValueFracLength=14  denProdOutputFracLength=30  denAccumFracLength=30  secondMemoryFracLength=15
  Out : Outport  VectorParamsAs1DForOutWhenUnconnected=off
  wires:
  In/1 -> Generated Filter Block/1
  Generated Filter Block/1 -> Out/1

== system lab4/Channel 8/Modulating Freq Filter ==
  In : Inport
  Generated Filter Block : dsparch4/Biquad Filter  Tag=BlockMethodSubSystem  FilterSource=Dialog parameters  CoeffSource=Specify via dialog  FilterObject=BQF  IIRFiltStruct=Direct form II  BiQuadCoeffs=[0.000543646210457578508 0 -0.000543646210457578508 1 -1.67915493521151493 0.999668262987304379;0.000362277711646738759 0 -0.000362277711646738759 1 -1.67853010478721987 0.999667968153815312;0.000383760550090824154 0 -0.000383760550090824154 1 -1.67865129764874688 0.999350908250753456;0.000311267935113039411 0 -0.000311267935113039411 1 -1.67850125802532069 0.999350769844989717;0.000383952786469986805 0 -0.000383952786469986805 1 -1.67888250518506932 0.999463216611433336;0.000138632850397095024 0 -0.000138632850397095024 1 -1.67845836248891178 0.999462892902345246;0.000561526906870492455 0 -0.000561526906870492455 1 -1.67942155864617071 0.999930643552372711;0.000222597052458937744 0 -0.000222597052458937744 1 -1.67870414971186932 0.999930572758238601;0.000526029046929657766 0 -0.000526029046929657766 1 -1.67901643278396584 0.999556046130124054;0.000385720749777551664 0 -0.000385720749777551664 1 -1.67848021797253089 0.999555707591358589;0.000332465712867440854 0 -0.000332465712867440854 1 -1.67856411401968297 0.999336341215274038;0.000382214506544261041 0 -0.000382214506544261041 1 -1.67875899629334757 0.99939382662440357;0.0001657983387453029 0 -0.0001657983387453029 1 -1.67846548317577016 0.999393573674031477;0.000555528362480964201 0 -0.000555528362480964201 1 -1.67929197006878583 0.999794971209438055;0.920679093800087722 0 -0.920679093800087722 1 -1.67860585071706714 0.999794771078190481]  ScaleValues=[0.000190628384599767972;1;1;1;1;1;1;1;1;1;1;1;1;1;1;1]  IC=0  ICnum=0  ICden=0  a0Flag=Warning  optimizeScaleValues=off  ScaleValueMode=Specify via input port (g)  roundingMode=Floor  overflowMode=off  scaleValueFracLength=14  denProdOutputFracLength=30  denAccumFracLength=30  secondMemoryFracLength=15
  Out : Outport  VectorParamsAs1DForOutWhenUnconnected=off
  wires:
  In/1 -> Generated Filter Block/1
  Generated Filter Block/1 -> Out/1

== system lab4/Channel 9/Modulating Freq Filter ==
  In : Inport
  Generated Filter Block : dsparch4/Biquad Filter  Tag=BlockMethodSubSystem  FilterSource=Dialog parameters  CoeffSource=Specify via dialog  FilterObject=BQF  IIRFiltStruct=Direct form II  BiQuadCoeffs=[0.000430884897719799786 0 -0.000430884897719799786 1 -1.65130895902990282 0.999668248904853729;0.000337909313595490402 0 -0.000337909313595490402 1 -1.65066005110284975 0.999667969722985106;0.000355783825648803374 0 -0.000355783825648803374 1 -1.65080058348771708 0.999350892347624531;0.000293361058718498067 0 -0.000293361058718498067 1 -1.65064476827856321 0.999350761276195598;0.00038206090425852129 0 -0.00038206090425852129 1 -1.65103550907129737 0.999463197897551892;0.000255724105188009161 0 -0.000255724105188009161 1 -1.65059503341199298 0.999462891373461781;0.000255808725244878422 0 -0.000255808725244878422 1 -1.65157372621484977 0.999930640369777635;0.000446362927787091572 0 -0.000446362927787091572 1 -1.65082864817862296 0.999930573324157357;0.000307307402905615437 0 -0.000307307402905615437 1 -1.65117030664944942 0.999556028773693539;0.00043477316052971984 0 -0.00043477316052971984 1 -1.65061343680282913 0.999555708203621607;0.000308661407291236387 0 -0.000308661407291236387 1 -1.6507107136818373 0.999336328706140309;0.000369764088881365883 0 -0.000369764088881365883 1 -1.65091044827969546 0.999393808466946809;0.000259995382328916471 0 -0.000259995382328916471 1 -1.65060563514024938 0.999393568974855651;0.000405667308834257718 0 -0.000405667308834257718 1 -1.6514454168974213 0.999794962030154277;0.886289684768096886 0 -0.886289684768096886 1 -1.65073284717045099 0.999794772522851427]  ScaleValues=[0.000270032776707598051;1;1;1;1;1;1;1;1;1;1;1;1;1;1;1]  IC=0  ICnum=0  ICden=0  a0Flag=Warning  optimizeScaleValues=off  ScaleValueMode=Specify via input port (g)  roundingMode=Floor  overflowMode=off  scaleValueFracLength=14  denProdOutputFracLength=30  denAccumFracLength=30  secondMemoryFracLength=15
  Out : Outport  VectorParamsAs1DForOutWhenUnconnected=off
  wires:
  In/1 -> Generated Filter Block/1
  Generated Filter Block/1 -> Out/1

== system lab4/Individual Signal Extractor/Modulating Freq Filter ==
  In : Inport
  Generated Filter Block : dsparch4/Biquad Filter  Tag=BlockMethodSubSystem  FilterSource=Dialog parameters  CoeffSource=Specify via dialog  FilterObject=BQF  IIRFiltStruct=Direct form II  BiQuadCoeffs=[0.000447834192739895044 0 -0.000447834192739895044 1 -1.84342145835843008 0.999668405594225651;0.000352702272994555224 0 -0.000352702272994555224 1 -1.84297530266396015 0.99966795227800076;0.000393389037410715866 0 -0.000393389037410715866 1 -1.84295972447575496 0.999351069372707124;0.000271522397118558259 0 -0.000271522397118558259 1 -1.84285253444748021 0.99935085656781808;0.000439928533426870458 0 -0.000439928533426870458 1 -1.8431609620298508 0.999463406116796627;0.000179968694146031232 0 -0.000179968694146031232 1 -1.8428580048816825 0.999462908410175377;0.000433029410195073577 0 -0.000433029410195073577 1 -1.84369625970029016 0.999930675836544713;0.000269558668079343837 0 -0.000269558668079343837 1 -1.8431842180074598 0.999930566975026469;0.000434295423850435938 0 -0.000434295423850435938 1 -1.84328645928743917 0.999556221907486164;0.000385090966757165032 0 -0.000385090966757165032 1 -1.84290350897479316 0.999555701394280849;0.000303547956367676715 0 -0.000303547956367676715 1 -1.8428927773742525 0.999336467904331727;0.000418382354530299778 0 -0.000418382354530299778 1 -1.84305044171901544 0.999394010334468064;0.000191838924433208831 0 -0.000191838924433208831 1 -1.8428407671553253 0.999393621449692682;0.00048034125864483652 0 -0.00048034125864483652 1 -1.84356007278210687 0.999795064162199099;1.28986266810011485 0 -1.28986266810011485 1 -1.84307025531527069 0.999794756459478462]  ScaleValues=[0.00016526438313770015;1;1;1;1;1;1;1;1;1;1;1;1;1;1;1]  IC=0  ICnum=0  ICden=0  a0Flag=Warning  optimizeScaleValues=off  ScaleValueMode=Specify via input port (g)  InputProcessing=Columns as channels (frame based)  roundingMode=Floor  overflowMode=off  scaleValueFracLength=14  denProdOutputFracLength=30  denAccumFracLength=30  secondMemoryFracLength=15
  Out : Outport  VectorParamsAs1DForOutWhenUnconnected=off
  wires:
  In/1 -> Generated Filter Block/1
  Generated Filter Block/1 -> Out/1
